simulink model "Simulacao_Robo"  (R2019a)
settings: Solver=FixedStepAuto  StartTime=0.0  StopTime=120  RelTol=1e-3
StopFcn:
  | figure,plot(out.tout,out.Theta);
  | hold on;
  | plot(out.tout,out.phi);
  | title('Ângulo de referência (Phi) e ângulo robô (Theta)');
  | xlabel('Tempo (s)');
  | ylabel('Angulos (rad)');
  | legend('Theta','Phi');
  | grid
  | 
  | figure,
  | subplot(2,1,1)
  | plot(out.tout,out.ed);
  | hold on;
  | plot(out.tout,out.ee);
  | xlabel('Tempo (s)');
  | ylabel('(a)');
  | grid
  | 
  | subplot(2,1,2),
  | plot(out.tout,out.etheta);
  | hold on;
  | plot(out.tout,out.es);
  | ylabel('(b)')
  | xlabel('Tempo (s)');
  | grid
  | 
  | figure,
  | plot(out.Xd,out.Yd);
  | hold on
  | plot(out.Xr,out.Yr);
  | grid
  | 
  | 
  | 
  | figure,plot(out.tout,out.X);hold on;plot(out.tout,out.Y);plot(out.tout,out.Theta);xlabel('Tempo[s]');legend('X','Y','Theta');grid
  | figure,plot(out.tout,out.Xd);hold on;plot(out.tout,out.Yd);hold on;xlabel('Tempo[s]');legend('Xd','Yd');grid
  | figure,plot(out.tout,out.s);hold on;plot(out.tout,out.s_ref);xlabel('Tempo[s]');legend('s','Theta');grid
  | figure,plot(out.tout,out.Ut);hold on;plot(out.tout,out.Ur);xlabel('Tempo[s]');legend('Sinal de Controle Linear','Sinal de Controle Rotacional');grid
  | 
  | 
  | 
  | 
  | 
  | 
  | figure
  | subplot(2,1,1);
  | plot(out.tout,out.X,out.tout,out.Xd,'.-');grid
  | subplot(2,1,2);
  | plot(out.tout,out.Y,out.tout,out.Yd,'.-');grid
values from neighbouring files (symbols this model uses):
  Kd_s = (2*zeta*Wn - B(1,1)) / B(1,1)    [Codigo_Controle_PID.m]
  Kd_t = (2*zeta*Wn - B(2,2)) / B(2,2)    [Codigo_Controle_PID.m]
  Kp_s = (Wn*Wn)/B(1,1)    [Codigo_Controle_PID.m]
  Kp_t = (Wn*Wn)/B(2,2)    [Codigo_Controle_PID.m]
libraries: simulink x3
settings Model: Creator=henri  LastModifiedBy=henri

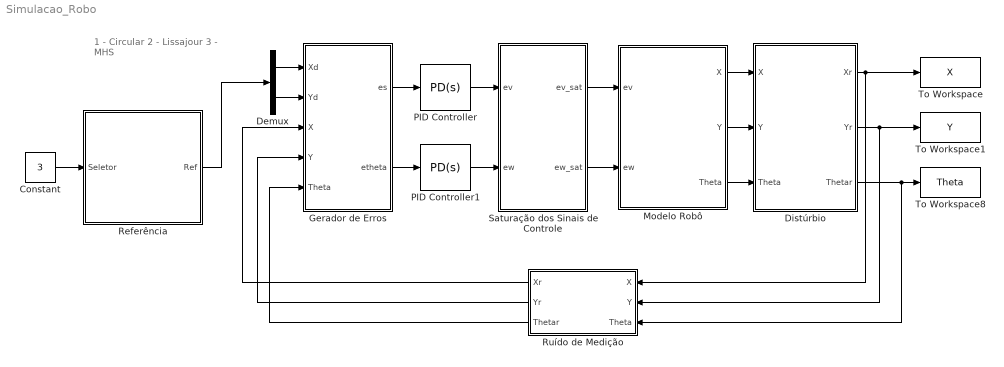
== system Simulacao_Robo ==
  note: 1 - Circular
      | 2 - Lissajour
      | 3 - MHS
  Constant : Constant  Value=3
  Demux : Demux  Outputs=2
  Distúrbio : Subsystem
  Gerador de Erros : Subsystem
  Modelo Robô : Subsystem
  PID Controller : simulink/Continuous/PID Controller  Controller=PD  Form=Parallel  TimeDomain=Continuous-time  SampleTime=-1  IntegratorMethod=Forward Euler  FilterMethod=Forward Euler  ControllerParametersSource=internal  P=Kp_s  I=0.01  D=Kd_s  UseFilter=on  N=5  TunerSelectOption=Transfer Function Based (PID Tuner App)  InitialConditionSource=internal  InitialConditionForIntegrator=0  InitialConditionForFilter=0  DifferentiatorICPrevScaledInput=0  ExternalReset=none  TrackingMode=off  Kt=1  LimitOutput=off  UpperSaturationLimit=inf  LowerSaturationLimit=-inf  LinearizeAsGain=on  AntiWindupMode=none  Kb=1  POutMin=[]  POutMax=[]  IOutMin=[]  IOutMax=[]  DOutMin=[]  DOutMax=[]  NOutMin=[]  NOutMax=[]  SumOutMin=[]  SumOutMax=[]  SaturationOutMin=[]  SaturationOutMax=[]  PParamMin=[]  PParamMax=[]  IParamMin=[]  IParamMax=[]  DParamMin=[]  DParamMax=[]  NParamMin=[]  NParamMax=[]  KbParamMin=[]  KbParamMax=[]  KtParamMin=[]  KtParamMax=[]  KbOutMin=[]  KbOutMax=[]  KtOutMin=[]  KtOutMax=[]  IntegratorOutMin=[]  IntegratorOutMax=[]  FilterOutMin=[]  FilterOutMax=[]  SumI1OutMin=[]  SumI1OutMax=[]  SumI2OutMin=[]  SumI2OutMax=[]  SumI3OutMin=[]  SumI3OutMax=[]  SumI4OutMin=[]  SumI4OutMax=[]  SumDOutMin=[]  SumDOutMax=[]  DifferentiatorOutMin=[]  DifferentiatorOutMax=[]  FilterDiffOutCoefMin=[]  FilterDiffOutCoefMax=[]  ReciprocalOutMin=[]  ReciprocalOutMax=[]  SumDenOutMin=[]  SumDenOutMax=[]  SumNumOutMin=[]  SumNumOutMax=[]  DivideOutMin=[]  DivideOutMax=[]  IntegratorContinuousStateAttributes=''  IntegratorStateMustResolveToSignalObject=off  IntegratorRTWStateStorageClass=Auto  FilterContinuousStateAttributes=''  FilterStateMustResolveToSignalObject=off  FilterRTWStateStorageClass=Auto  ParallelPVariant=InternalParameters  IdealPVariant=Disabled  IVariant=Disabled  DVariant=InternalParameters  IntegratorVariant=Disabled  SatVariant=Disabled  AWVariant=Disabled  PCopyVariant=Disabled  TRVariant=Disabled  FdbkBlocksVariant=Forward  IdealPFdbkVariant=Disabled  SatFdbkVariant=Disabled  DerivativeFilterVariant=ContFilter  NVariant=InternalParameters  NCopyVariant=Disabled  FilterICVariant=InternalICsFilter  IntegratorICVariant=Disabled  ExternalResetVariant=Disabled  TRSumVariant=Passthrough  SumFdbkVariant=Disabled  SumVariant=Sum_PD
  PID Controller1 : simulink/Continuous/PID Controller  Controller=PD  Form=Parallel  TimeDomain=Continuous-time  SampleTime=-1  IntegratorMethod=Forward Euler  FilterMethod=Forward Euler  ControllerParametersSource=internal  P=Kp_t  I=3.1  D=Kd_t  UseFilter=on  N=5  TunerSelectOption=Transfer Function Based (PID Tuner App)  InitialConditionSource=internal  InitialConditionForIntegrator=0  InitialConditionForFilter=0  DifferentiatorICPrevScaledInput=0  ExternalReset=none  TrackingMode=off  Kt=1  LimitOutput=off  UpperSaturationLimit=inf  LowerSaturationLimit=-inf  LinearizeAsGain=on  AntiWindupMode=none  Kb=1  POutMin=[]  POutMax=[]  IOutMin=[]  IOutMax=[]  DOutMin=[]  DOutMax=[]  NOutMin=[]  NOutMax=[]  SumOutMin=[]  SumOutMax=[]  SaturationOutMin=[]  SaturationOutMax=[]  PParamMin=[]  PParamMax=[]  IParamMin=[]  IParamMax=[]  DParamMin=[]  DParamMax=[]  NParamMin=[]  NParamMax=[]  KbParamMin=[]  KbParamMax=[]  KtParamMin=[]  KtParamMax=[]  KbOutMin=[]  KbOutMax=[]  KtOutMin=[]  KtOutMax=[]  IntegratorOutMin=[]  IntegratorOutMax=[]  FilterOutMin=[]  FilterOutMax=[]  SumI1OutMin=[]  SumI1OutMax=[]  SumI2OutMin=[]  SumI2OutMax=[]  SumI3OutMin=[]  SumI3OutMax=[]  SumI4OutMin=[]  SumI4OutMax=[]  SumDOutMin=[]  SumDOutMax=[]  DifferentiatorOutMin=[]  DifferentiatorOutMax=[]  FilterDiffOutCoefMin=[]  FilterDiffOutCoefMax=[]  ReciprocalOutMin=[]  ReciprocalOutMax=[]  SumDenOutMin=[]  SumDenOutMax=[]  SumNumOutMin=[]  SumNumOutMax=[]  DivideOutMin=[]  DivideOutMax=[]  IntegratorContinuousStateAttributes=''  IntegratorStateMustResolveToSignalObject=off  IntegratorRTWStateStorageClass=Auto  FilterContinuousStateAttributes=''  FilterStateMustResolveToSignalObject=off  FilterRTWStateStorageClass=Auto  ParallelPVariant=InternalParameters  IdealPVariant=Disabled  IVariant=Disabled  DVariant=InternalParameters  IntegratorVariant=Disabled  SatVariant=Disabled  AWVariant=Disabled  PCopyVariant=Disabled  TRVariant=Disabled  FdbkBlocksVariant=Forward  IdealPFdbkVariant=Disabled  SatFdbkVariant=Disabled  DerivativeFilterVariant=ContFilter  NVariant=InternalParameters  NCopyVariant=Disabled  FilterICVariant=InternalICsFilter  IntegratorICVariant=Disabled  ExternalResetVariant=Disabled  TRSumVariant=Passthrough  SumFdbkVariant=Disabled  SumVariant=Sum_PD
  Referência : Subsystem
  Ruído de Medição : Subsystem
  Saturação dos Sinais de Controle : Subsystem
  To Workspace : ToWorkspace  VariableName=X  SampleTime=-1
  To Workspace1 : ToWorkspace  VariableName=Y  SampleTime=-1
  To Workspace8 : ToWorkspace  VariableName=Theta  SampleTime=-1
  wires:
  Gerador de Erros/2(etheta) -> PID Controller1/1
  Demux/1 -> Gerador de Erros/1(Xd)
  Referência/1(Ref) -> Demux/1
  Gerador de Erros/1(es) -> PID Controller/1
  Demux/2 -> Gerador de Erros/2(Yd)
  Constant/1 -> Referência/1(Seletor)
  PID Controller/1 -> Saturação dos Sinais de Controle/1("ev ")
  PID Controller1/1 -> Saturação dos Sinais de Controle/2(ew)
  Modelo Robô/1(X) -> Distúrbio/1("X ")
  Modelo Robô/2(Y) -> Distúrbio/2(Y)
  Distúrbio/2(Yr) -> To Workspace1/1, Ruído de Medição/2(Y)
  Distúrbio/1(Xr) -> Ruído de Medição/1("X "), To Workspace/1
  Modelo Robô/3("Theta ") -> Distúrbio/3("Theta ")
  Distúrbio/3(Thetar) -> Ruído de Medição/3("Theta "), To Workspace8/1
  Saturação dos Sinais de Controle/1(ev_sat) -> Modelo Robô/1("ev ")
  Saturação dos Sinais de Controle/2(ew_sat) -> Modelo Robô/2(ew)
  Ruído de Medição/1(Xr) -> Gerador de Erros/3(X)
  Ruído de Medição/2(Yr) -> Gerador de Erros/4(Y)
  Ruído de Medição/3(Thetar) -> Gerador de Erros/5("Theta ")

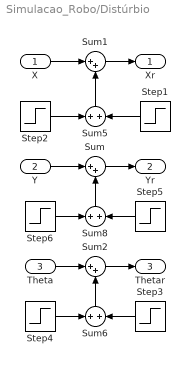
== system Simulacao_Robo/Distúrbio ==
  "X " : Inport
  Y : Inport  Port=2
  "Theta " : Inport  Port=3
  Step1 : Step  Time=60  After=0.03  SampleTime=0
  Step2 : Step  Time=61  After=-0.03  SampleTime=0
  Step3 : Step  Time=61  After=-0.5  SampleTime=0
  Step4 : Step  Time=60  After=0.5  SampleTime=0
  Step5 : Step  Time=60  After=-0.03  SampleTime=0
  Step6 : Step  Time=61  After=0.03  SampleTime=0
  Sum : Sum  Inputs=|++
  Sum1 : Sum  Inputs=|++
  Sum2 : Sum  Inputs=|++
  Sum5 : Sum  Inputs=+|+
  Sum6 : Sum  Inputs=+|+
  Sum8 : Sum  Inputs=+|+
  Xr : Outport
  Yr : Outport  Port=2
  Thetar : Outport  Port=3
  wires:
  "X "/1 -> Sum1/1
  Sum1/1 -> Xr/1
  Y/1 -> Sum/1
  Sum/1 -> Yr/1
  "Theta "/1 -> Sum2/1
  Sum2/1 -> Thetar/1
  Step2/1 -> Sum5/1
  Step1/1 -> Sum5/2
  Sum5/1 -> Sum1/2
  Step5/1 -> Sum8/2
  Step6/1 -> Sum8/1
  Sum8/1 -> Sum/2
  Step3/1 -> Sum6/2
  Step4/1 -> Sum6/1
  Sum6/1 -> Sum2/2

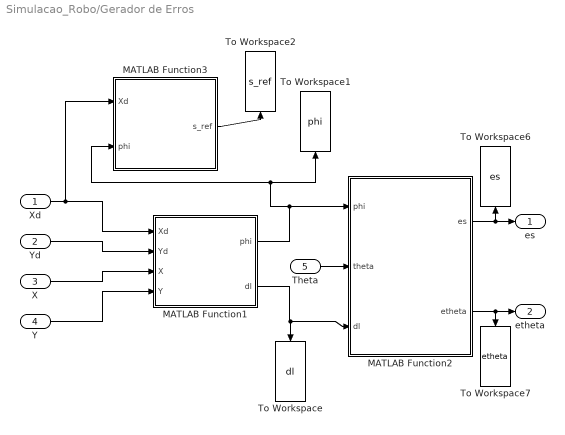
== system Simulacao_Robo/Gerador de Erros ==
  Xd : Inport
  Yd : Inport  Port=2
  X : Inport  Port=3
  Y : Inport  Port=4
  "Theta " : Inport  Port=5
  MATLAB Function1 : MATLAB Function  TreatAsAtomicUnit=on
  MATLAB Function2 : MATLAB Function  TreatAsAtomicUnit=on
  MATLAB Function3 : MATLAB Function  TreatAsAtomicUnit=on
  To Workspace : ToWorkspace  VariableName=dl  SampleTime=-1
  To Workspace1 : ToWorkspace  VariableName=phi  SampleTime=-1
  To Workspace2 : ToWorkspace  VariableName=s_ref  SampleTime=-1
  To Workspace6 : ToWorkspace  VariableName=es  SampleTime=-1
  To Workspace7 : ToWorkspace  VariableName=etheta  SampleTime=-1
  es : Outport
  etheta : Outport  Port=2
  wires:
  MATLAB Function1/1(phi) -> MATLAB Function2/1(phi), MATLAB Function3/2(phi), To Workspace1/1
  MATLAB Function1/2(dl) -> MATLAB Function2/3(dl), To Workspace/1
  MATLAB Function2/1(es) -> es/1, To Workspace6/1
  MATLAB Function2/2(etheta) -> etheta/1, To Workspace7/1
  "Theta "/1 -> MATLAB Function2/2(theta)
  Xd/1 -> MATLAB Function3/1(Xd), MATLAB Function1/1(Xd)
  Yd/1 -> MATLAB Function1/2(Yd)
  X/1 -> MATLAB Function1/3(X)
  Y/1 -> MATLAB Function1/4(Y)
  MATLAB Function3/1(s_ref) -> To Workspace2/1

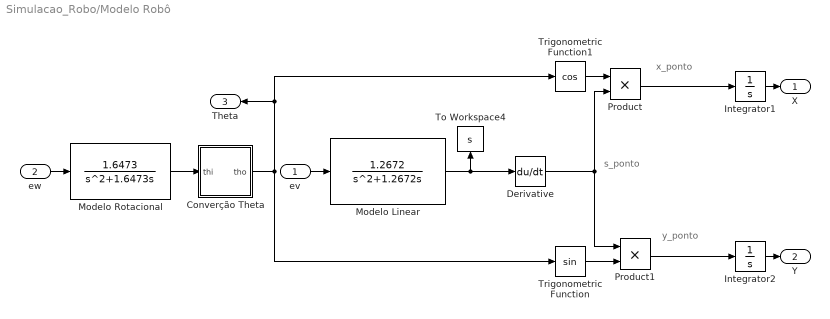
== system Simulacao_Robo/Modelo Robô ==
  note: s_ponto
  note: x_ponto
  note: y_ponto
  "ev " : Inport
  ew : Inport  Port=2
  Converção Theta : Subsystem
  Derivative : Derivative
  Integrator1 : Integrator
  Integrator2 : Integrator
  Modelo Linear : TransferFcn  Numerator=[1.2672]  Denominator=[1 1.2672 0]
  Modelo Rotacional : TransferFcn  Numerator=[1.6473]  Denominator=[1 1.6473 0]
  Product : Product
  Product1 : Product
  To Workspace4 : ToWorkspace  VariableName=s  SampleTime=-1
  Trigonometric Function : Trigonometry
  Trigonometric Function1 : Trigonometry  Operator=cos
  X : Outport
  Y : Outport  Port=2
  "Theta " : Outport  Port=3
  wires:
  Trigonometric Function/1 -> Product1/2
  Trigonometric Function1/1 -> Product/1
  Modelo Linear/1 -> Derivative/1, To Workspace4/1
  "ev "/1 -> Modelo Linear/1
  Product1/1 -> Integrator2/1
  Product/1 -> Integrator1/1
  ew/1 -> Modelo Rotacional/1
  Derivative/1 -> Product/2, Product1/1
  Integrator2/1 -> Y/1
  Integrator1/1 -> X/1
  Modelo Rotacional/1 -> Converção Theta/1("thi ")
  Converção Theta/1(tho) -> Trigonometric Function1/1, "Theta "/1, Trigonometric Function/1

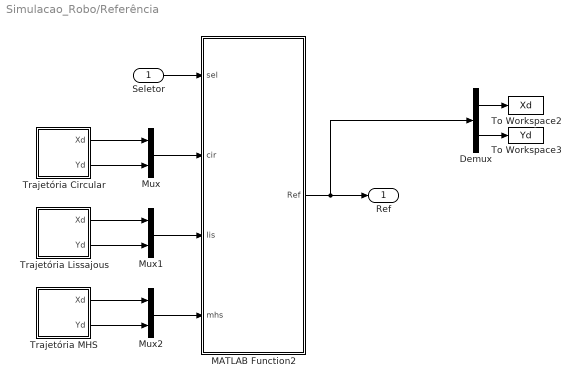
== system Simulacao_Robo/Referência ==
  Seletor : Inport
  Demux : Demux  Outputs=2
  MATLAB Function2 : MATLAB Function  TreatAsAtomicUnit=on
  Mux : Mux  Inputs=2
  Mux1 : Mux  Inputs=2
  Mux2 : Mux  Inputs=2
  To Workspace2 : ToWorkspace  VariableName=Xd  SampleTime=-1
  To Workspace3 : ToWorkspace  VariableName=Yd  SampleTime=-1
  Trajetória Circular : Subsystem
  Trajetória Lissajous : Subsystem
  Trajetória MHS : Subsystem
  Ref : Outport
  wires:
  Seletor/1 -> MATLAB Function2/1(sel)
  Trajetória Circular/2(Yd) -> Mux/2
  Trajetória Circular/1(Xd) -> Mux/1
  Mux/1 -> MATLAB Function2/2(cir)
  Trajetória Lissajous/1(Xd) -> Mux1/1
  Trajetória Lissajous/2(Yd) -> Mux1/2
  Mux1/1 -> MATLAB Function2/3(lis)
  Trajetória MHS/1(Xd) -> Mux2/1
  Trajetória MHS/2(Yd) -> Mux2/2
  Mux2/1 -> MATLAB Function2/4(mhs)
  MATLAB Function2/1(Ref) -> Ref/1, Demux/1
  Demux/2 -> To Workspace3/1
  Demux/1 -> To Workspace2/1

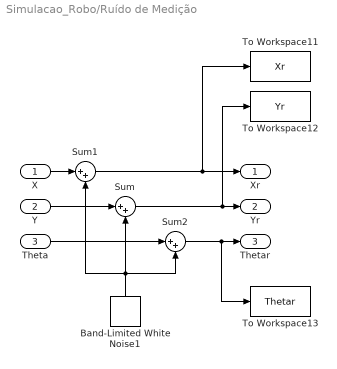
== system Simulacao_Robo/Ruído de Medição ==
  "X " : Inport
  Y : Inport  Port=2
  "Theta " : Inport  Port=3
  Band-Limited White Noise1 : simulink/Sources/Band-Limited White Noise  Cov=[0.00000005]  Ts=0.1  seed=[500000]
  Sum : Sum  Inputs=|++
  Sum1 : Sum  Inputs=|++
  Sum2 : Sum  Inputs=|++
  To Workspace11 : ToWorkspace  VariableName=Xr  SampleTime=-1
  To Workspace12 : ToWorkspace  VariableName=Yr  SampleTime=-1
  To Workspace13 : ToWorkspace  VariableName=Thetar  SampleTime=-1
  Xr : Outport
  Yr : Outport  Port=2
  Thetar : Outport  Port=3
  wires:
  Band-Limited White Noise1/1 -> Sum2/2, Sum/2, Sum1/2
  "X "/1 -> Sum1/1
  Sum1/1 -> To Workspace11/1, Xr/1
  Y/1 -> Sum/1
  Sum/1 -> To Workspace12/1, Yr/1
  "Theta "/1 -> Sum2/1
  Sum2/1 -> To Workspace13/1, Thetar/1

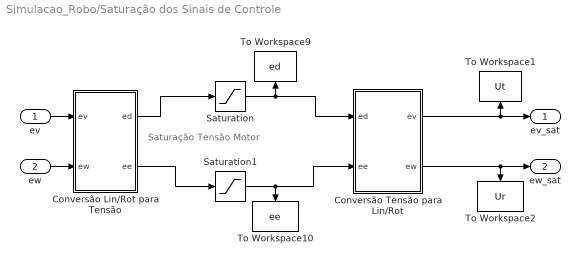
== system Simulacao_Robo/Saturação dos Sinais de Controle ==
  note: Saturação Tensão Motor
  "ev " : Inport
  ew : Inport  Port=2
  Conversão Lin/Rot para Tensão : MATLAB Function  TreatAsAtomicUnit=on
  "Conversão Tensão para Lin/Rot " : MATLAB Function  TreatAsAtomicUnit=on
  Saturation : Saturate  UpperLimit=6  LowerLimit=-6
  Saturation1 : Saturate  UpperLimit=6  LowerLimit=-6
  To Workspace1 : ToWorkspace  VariableName=Ut  SampleTime=-1
  To Workspace10 : ToWorkspace  VariableName=ee  SampleTime=-1
  To Workspace2 : ToWorkspace  VariableName=Ur  SampleTime=-1
  To Workspace9 : ToWorkspace  VariableName=ed  SampleTime=-1
  ev_sat : Outport
  ew_sat : Outport  Port=2
  wires:
  Conversão Lin/Rot para Tensão/2(ee) -> Saturation1/1
  "Conversão Tensão para Lin/Rot "/2(ew) -> ew_sat/1, To Workspace2/1
  "Conversão Tensão para Lin/Rot "/1(ev) -> To Workspace1/1, ev_sat/1
  Saturation1/1 -> To Workspace10/1, "Conversão Tensão para Lin/Rot "/2(ee)
  Saturation/1 -> "Conversão Tensão para Lin/Rot "/1(ed), To Workspace9/1
  Conversão Lin/Rot para Tensão/1(ed) -> Saturation/1
  "ev "/1 -> Conversão Lin/Rot para Tensão/1(ev)
  ew/1 -> Conversão Lin/Rot para Tensão/2(ew)

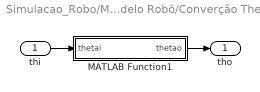
== system Simulacao_Robo/Modelo Robô/Converção Theta ==
  "thi " : Inport
  MATLAB Function1 : MATLAB Function  TreatAsAtomicUnit=on
  tho : Outport
  wires:
  "thi "/1 -> MATLAB Function1/1(thetai)
  MATLAB Function1/1(thetao) -> tho/1

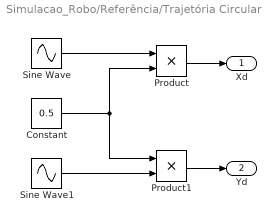
== system Simulacao_Robo/Referência/Trajetória Circular ==
  Constant : Constant  Value=0.5
  Product : Product
  Product1 : Product
  Sine Wave : Sin  Frequency=0.0625  Phase=pi/2  SampleTime=0
  Sine Wave1 : Sin  Frequency=0.0625  SampleTime=0
  Xd : Outport
  Yd : Outport  Port=2
  wires:
  Constant/1 -> Product/2, Product1/1
  Sine Wave/1 -> Product/1
  Sine Wave1/1 -> Product1/2
  Product/1 -> Xd/1
  Product1/1 -> Yd/1

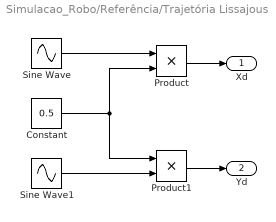
== system Simulacao_Robo/Referência/Trajetória Lissajous ==
  Constant : Constant  Value=0.5
  Product : Product
  Product1 : Product
  Sine Wave : Sin  Frequency=0.05  SampleTime=0
  Sine Wave1 : Sin  Frequency=0.1  SampleTime=0
  Xd : Outport
  Yd : Outport  Port=2
  wires:
  Constant/1 -> Product/2, Product1/1
  Sine Wave/1 -> Product/1
  Sine Wave1/1 -> Product1/2
  Product/1 -> Xd/1
  Product1/1 -> Yd/1

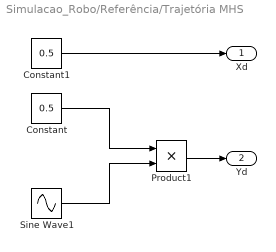
== system Simulacao_Robo/Referência/Trajetória MHS ==
  Constant : Constant  Value=0.5
  Constant1 : Constant  Value=0.5
  Product1 : Product
  Sine Wave1 : Sin  Frequency=0.1  SampleTime=0
  Xd : Outport
  Yd : Outport  Port=2
  wires:
  Constant/1 -> Product1/1
  Sine Wave1/1 -> Product1/2
  Product1/1 -> Yd/1
  Constant1/1 -> Xd/1

== matlab function Simulacao_Robo/Modelo Robô/Converção Theta/MATLAB Function1 ==
  data: thetai input; thetao output
%%%%%%%%%%%%%%%%%%%%%%%%%%%%%%%%%%%%%%%%%%%%%%%%%%
%%%%%%%%%%% CONVERSAO DE THETA %%%%%%%%%%%
%%%%%%%%%%%%%%%%%%%%%%%%%%%%%%%%%%%%%%%%%%%%%%%%%%

function thetao = fcn(thetai)

if(thetai >= 0) % VERIFICA SE O THETA DO ROBÔ É MAIOR QUE ZERO
    if((2*pi - thetai) < 0) % VERIFICA SE É MAIOR QUE 2PI
        thetai = 2*pi - thetai; % CONVERTE PARA O INTERVALO
        thetai = -thetai;       % DE 0 A 2PI
    end

    if((thetai <= pi) && (thetai >= 0)) % VERIFICA SE THETA ESTÁ EM PI >= THETA >= 0
        thetao = thetai; % MANTEM THETA NO INTERVALO
    else % THETA ESTÁ NO INTERVALO PI <= THETA <= 2PI
        thetao = thetai - 2*pi; % CONVERTE THETA PARA O INTERVALO -PI <= THETA <= 0
    end
else % THETA DO ROBÔ É MENOR QUE ZERO
   if((thetai >= -pi) && (thetai <= 0)) % VERIFICA SE THETA ESTÁ EM -PI <= THETA <= 0
        thetao = thetai; % MANTEM THETA NO INTERVALO
   else % THETA ESTÁ NO INTERVALO -PI >= THETA >= -2PI    
        thetao = thetai + 2*pi; % CONVERTE THETA PARA O INTERVALO PI >= THETA >= 0
    end   
end

== matlab function Simulacao_Robo/Gerador de Erros/MATLAB Function3 ==
  data: Xd input; s_ref output; phi input
%%%%%%%%%%%%%%%%%%%%%%%%%%%%%%%%%%%%%%%%%%%%%%%%%%
%%%%%%%%%%% FUNCAO CALCULO DE phi E dl %%%%%%%%%%%
%%%%%%%%%%%%%%%%%%%%%%%%%%%%%%%%%%%%%%%%%%%%%%%%%%

function s_ref  = fcn(Xd,phi)

s_ref = Xd / sin(phi);

end

== matlab function Simulacao_Robo/Gerador de Erros/MATLAB Function1 ==
  data: Xd input; phi output; Yd input; X input; Y input; dl output
%%%%%%%%%%%%%%%%%%%%%%%%%%%%%%%%%%%%%%%%%%%%%%%%%%
%%%%%%%%%%% FUNCAO CALCULO DE phi E dl %%%%%%%%%%%
%%%%%%%%%%%%%%%%%%%%%%%%%%%%%%%%%%%%%%%%%%%%%%%%%%

function [phi,dl] = fcn(Xd,Yd,X,Y)

phi = atan2((Yd-Y),(Xd-X)); % CALCULO DE PHI
dl = sqrt((Yd-Y)*(Yd-Y)+(Xd-X)*(Xd-X)); % CALCULO DE DL

end

== matlab function Simulacao_Robo/Gerador de Erros/MATLAB Function2 ==
  data: es output; phi input; etheta output; theta input; dl input
%%%%%%%%%%%%%%%%%%%%%%%%%%%%%%%%%%%%%%%%%%%%%%%%%%
%%%%%% CALCULO DOS ERROS LINEAR E ANGULAR %%%%%%%%
%%%%%%%%%%%%%%%%%%%%%%%%%%%%%%%%%%%%%%%%%%%%%%%%%%


function [es,etheta] = fcn(phi,theta,dl)

dphi = phi-theta;

es = dl*cos(phi-theta); % ERRO LINEAR

    if(abs(dphi) < pi/2) % ERRO ANGULAR
        etheta = dphi;
        %etheta = sin(etheta);
    else
        etheta = dphi - pi*sign(dphi);
        %etheta = sin(etheta);
    end
end

== matlab function Simulacao_Robo/Referência/MATLAB Function2 ==
  data: Ref output; sel input; cir input; lis input; mhs input
%%%%%%%%%%%%%%%%%%%%%%%%%%%%%%%%%%%%%%%%%%%%%%%%%%
%%%%%%%%%%%%%% SELECAO DE TRAJETORIA %%%%%%%%%%%%%
%%%%%%%%%%%%%%%%%%%%%%%%%%%%%%%%%%%%%%%%%%%%%%%%%%

function Ref = fcn(sel,cir,lis,mhs)

if(sel == 1)        % SELECIONA CIRCULAR
    Ref = cir;
elseif(sel == 2)    % SELECIONA CURVA DE BERNOULLI
    Ref = lis;
else                % ESTRATEGIA DE DEFESA MHS
    Ref = mhs;
end

== matlab function Simulacao_Robo/Saturação dos Sinais de Controle/Conversão Lin//Rot para Tensão ==
  data: ev input; ed output; ew input; ee output
%%%%%%%%%%%%%%%%%%%%%%%%%%%%%%%%%%%%%%%%%%%%%%%%%%
%%%%%% CONVERSAO LIN/ROT -> TENSAO MOTORES %%%%%%%
%%%%%%%%%%%%%%%%%%%%%%%%%%%%%%%%%%%%%%%%%%%%%%%%%%

function [ed,ee] = fcn(ev,ew)

ed = 20.0973*ev + 0.1529*ew; % TENSAO MOTOR DIREITO
ee = 20.0973*ev - 0.1529*ew; % TENSÃO MOTOR ESQUERDO

== matlab function Simulacao_Robo/Saturação dos Sinais de Controle/Conversão Tensão para Lin//Rot  ==
  data: ed input; ev output; ee input; ew output
%%%%%%%%%%%%%%%%%%%%%%%%%%%%%%%%%%%%%%%%%%%%%%%%%%
%%%%%% CONVERSAO TENSAO MOTORES -> LIN/ROT %%%%%%%
%%%%%%%%%%%%%%%%%%%%%%%%%%%%%%%%%%%%%%%%%%%%%%%%%%

function [ev,ew] = fcn(ed,ee)

ev = 0.0249*ed + 0.0249*ee; % SINAL CONTROLE LINEAR
ew = 3.2695*ed - 3.2695*ee; % SINAL CONTROLE ROTACIONAL
